simulink model "Model_SD_CIFB_k2_TC_param"  (R2023b)
settings: Solver=ode45  StartTime=0.0  StopTime=Tstop  RelTol=1e-3  EnableMultiTasking=on
values from neighbouring files (symbols this model uses):
  A1 = 10000    [run_Model_SD_CIFB_k2.m]
  A2 = A1    (= 10000)    [run_Model_SD_CIFB_k2.m]
  Amp = 10^(Av/20)*FS    (= 0.501187233627)    [run_Model_SD_CIFB_k2.m]
  C = 100e-12    (= 1e-10)    [run_Model_SD_CIFB_k2.m]
  fs = 2*BA*OSR    (= 2560000)    [run_Model_SD_CIFB_k2.m]
  OSR = 64    [run_Model_SD_CIFB_k2.m]
  R11 = 1/(a1*fs*C)    (= 11718.75)    [run_Model_SD_CIFB_k2.m]
  R22 = 1/(a2*fs*C)    (= 1302.08333333)    [run_Model_SD_CIFB_k2.m]
  tau = A1/GBW    (= 0.0002)    [run_Model_SD_CIFB_k2.m]
  ts = 1/fs    (= 3.90625e-07)    [run_Model_SD_CIFB_k2.m]
  win = 2*pi*fin    [run_Model_SD_CIFB_k2.m]
undefined symbols (not defined in the file or in its folder): R21, tau2
settings Model: Creator=cellierr  LastModifiedBy=martincova
settings SolverCC: AlgebraicLoopSolver=TrustRegion
settings DataIOCC: LimitDataPoints=on  SaveFormat=Array  ReturnWorkspaceOutputs=off
settings OptimizationCC: ExpressionDepthLimit=2147483647  InitFltsAndDblsToZero=on  LifeSpan=inf
settings DebuggingCC: SaveWithParameterizedLinksMsg=none  UnderspecifiedInitializationDetection=Classic  MergeDetectMultiDrivingBlocksExec=none  SolverPrmCheckMsg=warning  FcnCallInpInsideContextMsg=warning  UnconnectedInputMsg=warning  UnconnectedOutputMsg=warning  UnconnectedLineMsg=warning  StateNameClashWarn=warning  SFUnexpectedBacktrackingDiag=warning  SFNoUnconditionalDefaultTransitionDiag=warning  SFExecutionAtInitializationDiag=none  ArithmeticOperatorsInVariantConditions=warning
settings HardwareCC: ProdBitPerPointer=32  ProdBitPerSizeT=32  ProdBitPerPtrDiffT=32  ProdLargestAtomicFloat=None  ProdIntDivRoundTo=Undefined  ProdEndianess=Unspecified  ProdWordSize=32  ProdHWDeviceType=32-bit Generic
settings ModelReferenceCC: EnableRefExpFcnMdlSchedulingChecks=on  PropagateSignalLabelsOutOfModel=off
settings SFSimCC: SimUseLocalCustomCode=off  CustomCodeUndefinedFunction=UseInterfaceOnly
settings RTWCC: RTWUseLocalCustomCode=off
settings CodeAppCC: StateflowObjectComments=on
settings GRTTargetCC: TargetFcnLib=ansi_tfl_tmw.mat  TargetLangStandard=C89/C90 (ANSI)  CombineOutputUpdateFcns=off  GRTInterface=on
settings ConfigComp: CovMetricSettings=dw  CovSaveCumulativeToWorkspaceVar=on  CovSaveSingleToWorkspaceVar=on  CovExternalEMLEnable=off  CovSFcnEnable=off

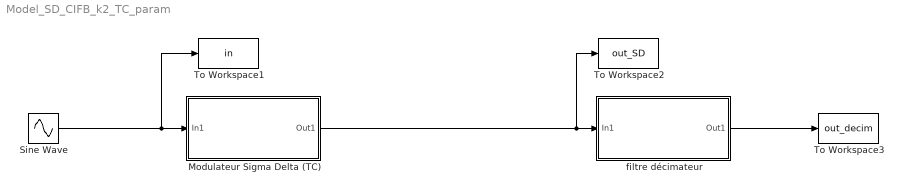
== system Model_SD_CIFB_k2_TC_param ==
  Modulateur Sigma Delta (TC) : Subsystem
  Sine Wave : Sin  Amplitude=Amp  Frequency=win  SampleTime=0
  To Workspace1 : ToWorkspace  VariableName=in  SampleTime=1/fs
  To Workspace2 : ToWorkspace  VariableName=out_SD  SampleTime=-1
  To Workspace3 : ToWorkspace  VariableName=out_decim  SampleTime=ts
  filtre décimateur : Subsystem
  wires:
  Sine Wave/1 -> To Workspace1/1, Modulateur Sigma Delta (TC)/1(In1)
  filtre décimateur/1(Out1) -> To Workspace3/1
  Modulateur Sigma Delta (TC)/1(Out1) -> filtre décimateur/1(In1), To Workspace2/1

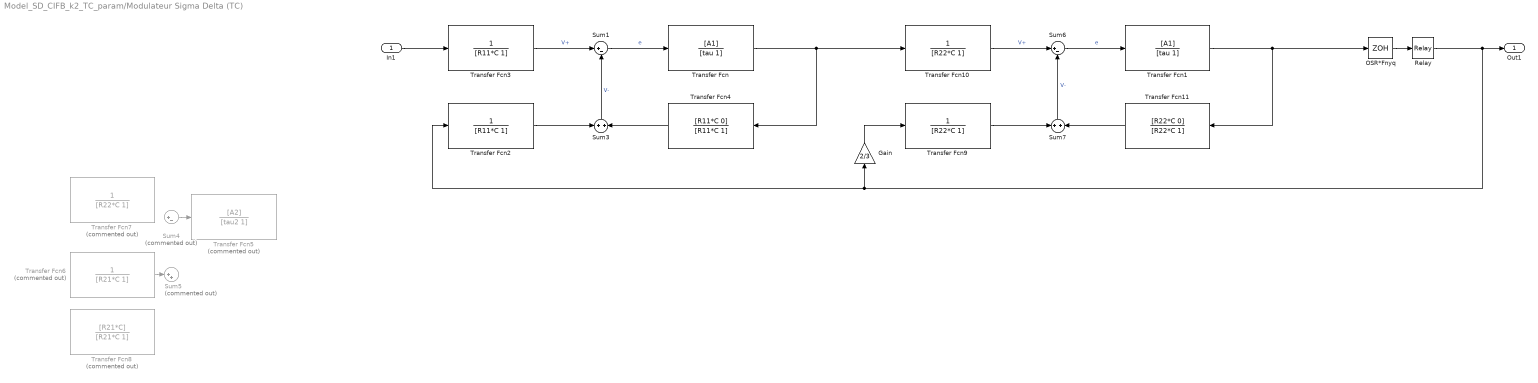
== system Model_SD_CIFB_k2_TC_param/Modulateur Sigma Delta (TC) ==
  In1 : Inport
  Gain : Gain  Gain=2/3
  OSR*Fnyq : ZeroOrderHold  SampleTime=1/(fs)
  Relay : Relay  OnSwitchValue=0  OffSwitchValue=0  OffOutputValue=-1
  Sum1 : Sum  Inputs=|+-
  Sum3 : Sum
  Sum4 : Sum  Commented=on  Inputs=|+-
  Sum5 : Sum  Commented=on  Inputs=|++
  Sum6 : Sum  Inputs=|+-
  Sum7 : Sum
  Transfer Fcn : TransferFcn  Numerator=[A1]  Denominator=[tau 1]
  Transfer Fcn1 : TransferFcn  Numerator=[A1]  Denominator=[tau 1]
  Transfer Fcn10 : TransferFcn  Denominator=[R22*C 1]
  Transfer Fcn11 : TransferFcn  Numerator=[R22*C 0]  Denominator=[R22*C 1]
  Transfer Fcn2 : TransferFcn  Denominator=[R11*C 1]
  Transfer Fcn3 : TransferFcn  Denominator=[R11*C 1]
  Transfer Fcn4 : TransferFcn  Numerator=[R11*C 0]  Denominator=[R11*C 1]
  Transfer Fcn5 : TransferFcn  Commented=on  Numerator=[A2]  Denominator=[tau2 1]
  Transfer Fcn6 : TransferFcn  Commented=on  Denominator=[R21*C 1]
  Transfer Fcn7 : TransferFcn  Commented=on  Denominator=[R22*C 1]
  Transfer Fcn8 : TransferFcn  Commented=on  Numerator=[R21*C]  Denominator=[R21*C 1]
  Transfer Fcn9 : TransferFcn  Denominator=[R22*C 1]
  Out1 : Outport
  wires:
  OSR*Fnyq/1 -> Relay/1
  Transfer Fcn3/1 -> Sum1/1  "V+"
  Sum1/1 -> Transfer Fcn/1  "e"
  Transfer Fcn2/1 -> Sum3/1
  Sum3/1 -> Sum1/2  "V-"
  Transfer Fcn6/1 -> Sum5/1
  Sum4/1 -> Transfer Fcn5/1
  In1/1 -> Transfer Fcn3/1
  Transfer Fcn4/1 -> Sum3/2
  Relay/1 -> Gain/1, Transfer Fcn2/1, Out1/1
  Transfer Fcn9/1 -> Sum7/1
  Transfer Fcn1/1 -> OSR*Fnyq/1, Transfer Fcn11/1
  Sum6/1 -> Transfer Fcn1/1  "e"
  Sum7/1 -> Sum6/2  "V-"
  Transfer Fcn10/1 -> Sum6/1  "V+"
  Transfer Fcn11/1 -> Sum7/2
  Transfer Fcn/1 -> Transfer Fcn10/1, Transfer Fcn4/1
  Gain/1 -> Transfer Fcn9/1

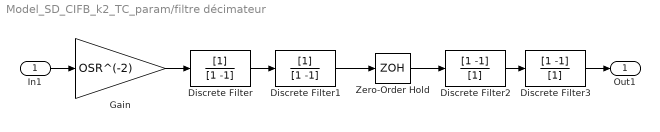
== system Model_SD_CIFB_k2_TC_param/filtre décimateur ==
  In1 : Inport
  Discrete Filter : DiscreteFilter  Denominator=[1 -1]
  Discrete Filter1 : DiscreteFilter  Denominator=[1 -1]
  Discrete Filter2 : DiscreteFilter  Numerator=[1 -1]  Denominator=[1]  SampleTime=ts*OSR
  Discrete Filter3 : DiscreteFilter  Numerator=[1 -1]  Denominator=[1]  SampleTime=ts*OSR
  Gain : Gain  Gain=OSR^(-2)  SaturateOnIntegerOverflow=on  OutDataTypeStr=Inherit: Same as input  ParamDataTypeStr=Inherit: Same as input
  Zero-Order Hold : ZeroOrderHold  SampleTime=ts*OSR
  Out1 : Outport
  wires:
  In1/1 -> Gain/1
  Discrete Filter3/1 -> Out1/1
  Gain/1 -> Discrete Filter/1
  Discrete Filter/1 -> Discrete Filter1/1
  Discrete Filter2/1 -> Discrete Filter3/1
  Discrete Filter1/1 -> Zero-Order Hold/1
  Zero-Order Hold/1 -> Discrete Filter2/1
